simulink model "P7"  (R2020b)
settings: Solver=VariableStepAuto  StartTime=0.0  StopTime=10.0  RelTol=1e-3
settings Model: Creator=stank  LastModifiedBy=stank

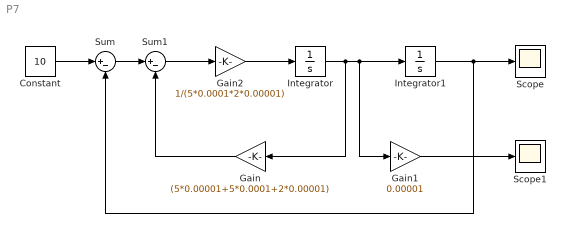
== system P7 ==
  Constant : Constant  Value=10
  Gain : Gain  Gain=(5*0.00001+5*0.0001+2*0.00001)
  Gain1 : Gain  Gain=0.00001
  Gain2 : Gain  Gain=1/(5*0.0001*2*0.00001)
  Integrator : Integrator
  Integrator1 : Integrator
  Scope : Scope
  Scope1 : Scope
  Sum : Sum  Inputs=|+-
  Sum1 : Sum  Inputs=|+-
  wires:
  Constant/1 -> Sum/1
  Sum/1 -> Sum1/1
  Integrator/1 -> Gain/1, Gain1/1, Integrator1/1
  Gain1/1 -> Scope1/1
  Integrator1/1 -> Sum/2, Scope/1
  Gain/1 -> Sum1/2
  Sum1/1 -> Gain2/1
  Gain2/1 -> Integrator/1
